simulink model "transmitter"  (R2021b)
settings: Solver=VariableStepAuto  StartTime=0.0  StopTime=200/100e3  RelTol=1e-3
PreLoadFcn:
  | setup_transmitter
InitFcn:
  | setup_transmitter
values from neighbouring files (symbols this model uses):
  tx_data = fi(double('Hello World!'), 0, 8, 0)    [setup_transmitter.m]
undefined symbols (not defined in the file or in its folder): AXI4, Lite, xlfda_numerator
libraries: hdlBasic x106, hdlsllib x6, hdlDSPIP x3, simulink x1, hdlUtilities x1, vmcUtilities x1
(part 2 of 2)

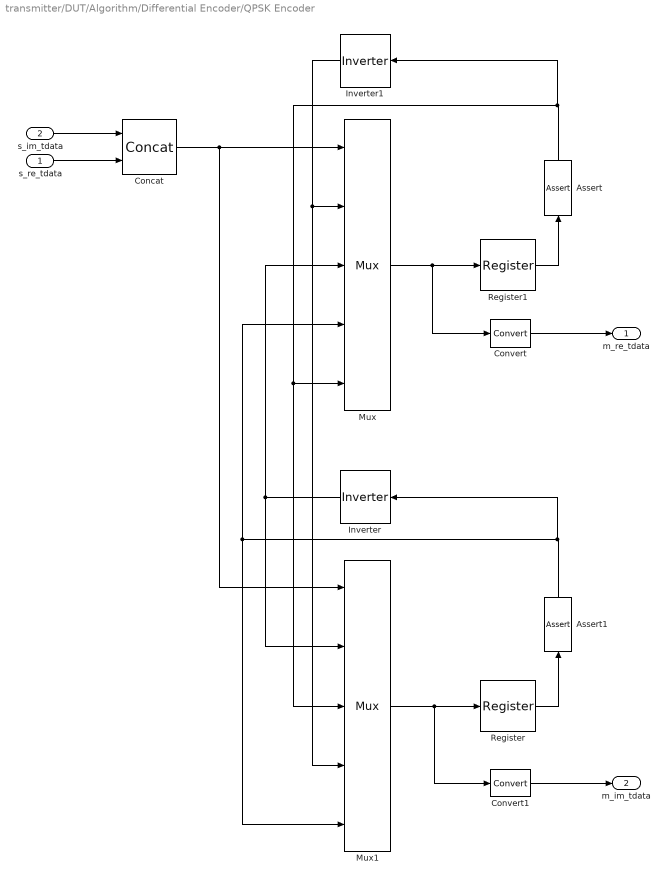
== system transmitter/DUT/Algorithm/Differential Encoder/QPSK Encoder ==
  s_re_tdata : Inport
  s_im_tdata : Inport  Port=2
  Assert : hdlBasic/Assert  assert_type=on  type_source=Explicitly  gui_display_data_type=Boolean  arith_type=Boolean  n_bits=16  bin_pt=14  preci_type=Single  exp_width=8  frac_width=24  assert_rate=off  rate_source=Explicitly  period=1  output_port=on  XmcBlockStatus=1  maskContainerNames=group1  block_type=assert  block_config=sysgen:assert_config  block_width=609  block_height=900
  Assert1 : hdlBasic/Assert  assert_type=on  type_source=Explicitly  gui_display_data_type=Boolean  arith_type=Boolean  n_bits=16  bin_pt=14  preci_type=Single  exp_width=8  frac_width=24  assert_rate=off  rate_source=Explicitly  period=1  output_port=on  XmcBlockStatus=1  maskContainerNames=group1  block_type=assert  block_config=sysgen:assert_config  block_width=609  block_height=900
  Concat : hdlBasic/Concat  num_inputs=2  XmcBlockStatus=1  maskContainerNames=group1  block_type=concat  block_config=sysgen:Concat_config
  Convert : hdlBasic/Convert  gui_display_data_type=Fixed-point  arith_type=Unsigned  n_bits=1  bin_pt=0  float_type=Single  exp_bits=8  fraction_bits=24  quantization=Truncate  overflow=Wrap  en=off  latency=0  pipeline=off  XmcBlockStatus=1  maskContainerNames=group2  block_type=convert  block_config=sysgen:Convert_config  block_width=595  block_height=885
  Convert1 : hdlBasic/Convert  gui_display_data_type=Fixed-point  arith_type=Unsigned  n_bits=1  bin_pt=0  float_type=Single  exp_bits=8  fraction_bits=24  quantization=Truncate  overflow=Wrap  en=off  latency=0  pipeline=off  XmcBlockStatus=1  maskContainerNames=group2  block_type=convert  block_config=sysgen:Convert_config  block_width=595  block_height=885
  Inverter : hdlBasic/Inverter  en=off  latency=0  XmcBlockStatus=1  maskContainerNames=group2  block_type=inv  block_config=sysgen:Inverter_config
  Inverter1 : hdlBasic/Inverter  en=off  latency=0  XmcBlockStatus=1  maskContainerNames=group2  block_type=inv  block_config=sysgen:Inverter_config
  Mux : hdlBasic/Mux  inputs=4  en=off  latency=0  precision=Full  arith_type=Unsigned  n_bits=16  bin_pt=14  quantization=Truncate  overflow=Wrap  XmcBlockStatus=1  maskContainerNames=tabcontainer1  block_type=mux  block_config=sysgen:Mux_config
  Mux1 : hdlBasic/Mux  inputs=4  en=off  latency=0  precision=Full  arith_type=Unsigned  n_bits=16  bin_pt=14  quantization=Truncate  overflow=Wrap  XmcBlockStatus=1  maskContainerNames=tabcontainer1  block_type=mux  block_config=sysgen:Mux_config
  Register : hdlBasic/Register  init=0  rst=off  en=off  XmcBlockStatus=1  maskContainerNames=tabcontainer1  block_type=register  block_config=sysgen:Register_config
  Register1 : hdlBasic/Register  init=0  rst=off  en=off  XmcBlockStatus=1  maskContainerNames=tabcontainer1  block_type=register  block_config=sysgen:Register_config
  m_re_tdata : Outport
  m_im_tdata : Outport  Port=2
  wires:
  s_im_tdata/1 -> Concat/1
  s_re_tdata/1 -> Concat/2
  Mux1/1 -> Convert1/1, Register/1
  Mux/1 -> Convert/1, Register1/1
  Register1/1 -> Assert/1
  Register/1 -> Assert1/1
  Inverter/1 -> Mux1/2, Mux/3
  Inverter1/1 -> Mux1/4, Mux/2
  Assert/1 -> Mux1/3, Mux/5, Inverter1/1
  Assert1/1 -> Mux/4, Mux1/5, Inverter/1
  Convert/1 -> m_re_tdata/1
  Convert1/1 -> m_im_tdata/1
  Concat/1 -> Mux1/1, Mux/1

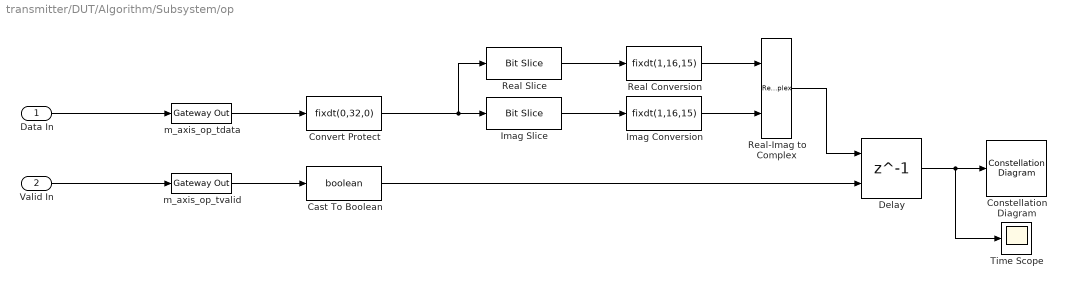
== system transmitter/DUT/Algorithm/Subsystem/op ==
  Data In : Inport
  Valid In : Inport  Port=2
  Cast To Boolean : DataTypeConversion  OutDataTypeStr=boolean
  Constellation Diagram : ConstellationDiagram
  Convert Protect : DataTypeConversion  OutDataTypeStr=fixdt(0,32,0)  ConvertRealWorld=Stored Integer (SI)
  Delay : Delay  DelayLength=1  ShowEnablePort=on
      settings: InputPortMap=u0,e6
  Imag Conversion : DataTypeConversion  OutDataTypeStr=fixdt(1,16,15)  ConvertRealWorld=Stored Integer (SI)
  Imag Slice : hdlsllib/Logic and Bit Operations/Bit Slice  lidx=31  ridx=16
      settings: SourceProductBaseCode=SL
  Real Conversion : DataTypeConversion  OutDataTypeStr=fixdt(1,16,15)  ConvertRealWorld=Stored Integer (SI)
  Real Slice : hdlsllib/Logic and Bit Operations/Bit Slice  lidx=15  ridx=0
      settings: SourceProductBaseCode=SL
  Real-Imag to Complex : RealImagToComplex
  Time Scope : Scope
  m_axis_op_tdata : hdlBasic/Gateway Out  inherit_from_input=on  hdl_port=on  rows=1  columns=1  UseAsDAC=off  DACChannel='1'  interface=None  automatic_assignment=on  address_offset=hex2dec('00')  intf_name=''  intf_description=''  timing_constraint=None  locs_specified=off  LOCs={}  io_standard={}  XmcBlockStatus=1  maskContainerNames=group4  block_type=gatewayout  block_config=sysgen:gateway_out_config  block_width_w=590  block_height_w=620  block_width=620  block_height=750
  m_axis_op_tvalid : hdlBasic/Gateway Out  inherit_from_input=on  hdl_port=on  rows=1  columns=1  UseAsDAC=off  DACChannel='1'  interface=None  automatic_assignment=on  address_offset=hex2dec('00')  intf_name=''  intf_description=''  timing_constraint=None  locs_specified=off  LOCs={}  io_standard={}  XmcBlockStatus=1  maskContainerNames=group4  block_type=gatewayout  block_config=sysgen:gateway_out_config  block_width_w=590  block_height_w=620  block_width=620  block_height=750
  wires:
  Valid In/1 -> m_axis_op_tvalid/1
  Data In/1 -> m_axis_op_tdata/1
  Delay/1 -> Time Scope/1, Constellation Diagram/1
  m_axis_op_tvalid/1 -> Cast To Boolean/1
  Real Conversion/1 -> Real-Imag to Complex/1
  Real Slice/1 -> Real Conversion/1
  Imag Slice/1 -> Imag Conversion/1
  Imag Conversion/1 -> Real-Imag to Complex/2
  m_axis_op_tdata/1 -> Convert Protect/1
  Real-Imag to Complex/1 -> Delay/1
  Convert Protect/1 -> Real Slice/1, Imag Slice/1
  Cast To Boolean/1 -> Delay/2
